simulink model "c2d_controller_continuous"  (R2015a)
settings: Solver=ode45  StartTime=0.0  StopTime=20  FixedStep=0.01  RelTol=1e-3
values from neighbouring files (symbols this model uses):
  Gcs = tf(40)    [c2d_controller_m.m]
  Gs = 1.0 / (s * s + 5 * s + 1)    [c2d_controller_m.m]
settings Model: Creator=Xiaotian  LastModifiedBy=Xiaotian

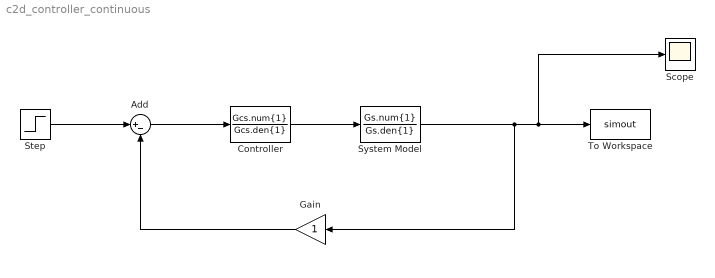
== system c2d_controller_continuous ==
  Add : Sum  Inputs=|+-
  Controller : TransferFcn  Numerator=Gcs.num{1}  Denominator=Gcs.den{1}
  Gain : Gain
  Scope : Scope
  Step : Step  SampleTime=0
  System Model : TransferFcn  Numerator=Gs.num{1}  Denominator=Gs.den{1}
  To Workspace : ToWorkspace  VariableName=simout  SaveFormat=Timeseries  SampleTime=0.1
  wires:
  Step/1 -> Add/1
  Gain/1 -> Add/2
  Add/1 -> Controller/1
  System Model/1 -> Gain/1, To Workspace/1, Scope/1
  Controller/1 -> System Model/1
